simulink model "DZ_AC_ol"  (R2019b)
settings: Solver=VariableStepAuto  StartTime=0.0  StopTime=1  RelTol=1e-3
undefined symbols (not defined in the file): alfa_beta, beta, j, J, Lkm, Lks, np, omega, rad_to_rpm, Rr, Rs, T_1_amp, T_amp, Vmax
libraries: simulink x3
settings Model: Creator=denni  LastModifiedBy=denniszanutto

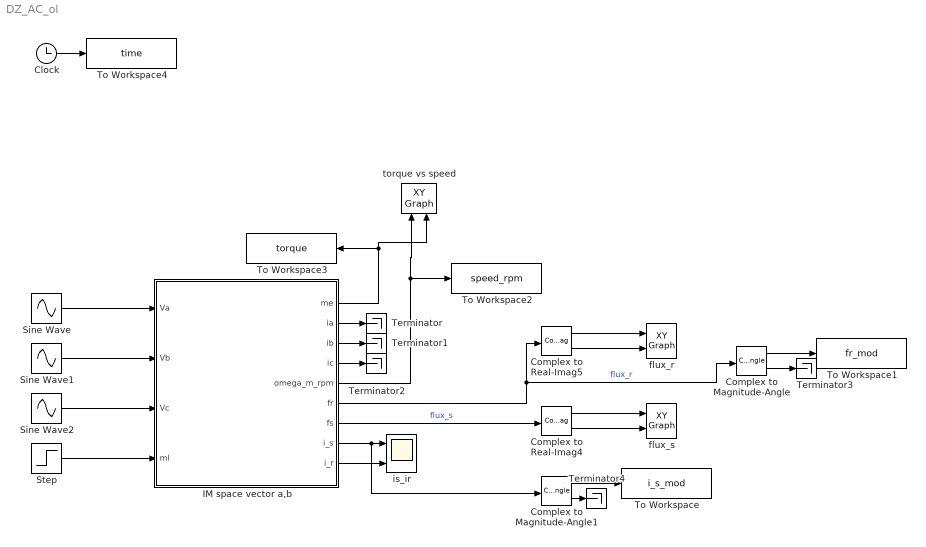
== system DZ_AC_ol ==
  Clock : Clock
  Complex to Magnitude-Angle : ComplexToMagnitudeAngle
  Complex to Magnitude-Angle1 : ComplexToMagnitudeAngle
  Complex to Real-Imag4 : ComplexToRealImag
  Complex to Real-Imag5 : ComplexToRealImag
  IM space vector a,b : Subsystem
  Sine Wave : Sin  Amplitude=Vmax  Frequency=omega  SampleTime=0
  Sine Wave1 : Sin  Amplitude=Vmax  Frequency=omega  Phase=-2*pi/3  SampleTime=0
  Sine Wave2 : Sin  Amplitude=Vmax  Frequency=omega  Phase=2*pi/3  SampleTime=0
  Step : Step  Time=0  After=0  SampleTime=0
  Terminator{,1..4} (5 alike) : Terminator
  To Workspace : ToWorkspace  VariableName=i_s_mod  SaveFormat=Timeseries  SampleTime=-1
  To Workspace1 : ToWorkspace  VariableName=fr_mod  SaveFormat=Timeseries  SampleTime=-1
  To Workspace2 : ToWorkspace  VariableName=speed_rpm  SaveFormat=Timeseries  SampleTime=-1
  To Workspace3 : ToWorkspace  VariableName=torque  SaveFormat=Timeseries  SampleTime=-1
  To Workspace4 : ToWorkspace  VariableName=time  SaveFormat=Timeseries  SampleTime=-1
  flux_r : simulink/Sinks/XY Graph  xmin=-3  xmax=3  ymin=-3  ymax=3  st=-1
  flux_s : simulink/Sinks/XY Graph  xmin=-3  xmax=3  ymin=-3  ymax=3  st=-1
  is_ir : Scope  NumInputPorts=2
  torque vs speed : simulink/Sinks/XY Graph  xmin=0  xmax=1300  ymin=-800  ymax=1200  st=-1
  wires:
  Step/1 -> IM space vector a,b/4(ml)
  Sine Wave/1 -> IM space vector a,b/1(Va)
  Sine Wave1/1 -> IM space vector a,b/2(Vb)
  Sine Wave2/1 -> IM space vector a,b/3(Vc)
  Complex to Real-Imag4/2 -> flux_s/2
  IM space vector a,b/7(fs) -> Complex to Real-Imag4/1  "flux_s"
  Complex to Real-Imag4/1 -> flux_s/1
  Complex to Real-Imag5/1 -> flux_r/1
  IM space vector a,b/6(fr) -> Complex to Real-Imag5/1, Complex to Magnitude-Angle/1  "flux_r"
  Complex to Real-Imag5/2 -> flux_r/2
  Complex to Magnitude-Angle/1 -> To Workspace1/1
  IM space vector a,b/8(i_s) -> Complex to Magnitude-Angle1/1, is_ir/1
  IM space vector a,b/9(i_r) -> is_ir/2
  IM space vector a,b/2(ia) -> Terminator/1
  IM space vector a,b/3(ib) -> Terminator1/1
  IM space vector a,b/4(ic) -> Terminator2/1
  IM space vector a,b/1("me ") -> torque vs speed/2, To Workspace3/1
  IM space vector a,b/5("omega_m_rpm ") -> To Workspace2/1, torque vs speed/1
  Complex to Magnitude-Angle/2 -> Terminator3/1
  Complex to Magnitude-Angle1/1 -> To Workspace/1
  Complex to Magnitude-Angle1/2 -> Terminator4/1
  Clock/1 -> To Workspace4/1

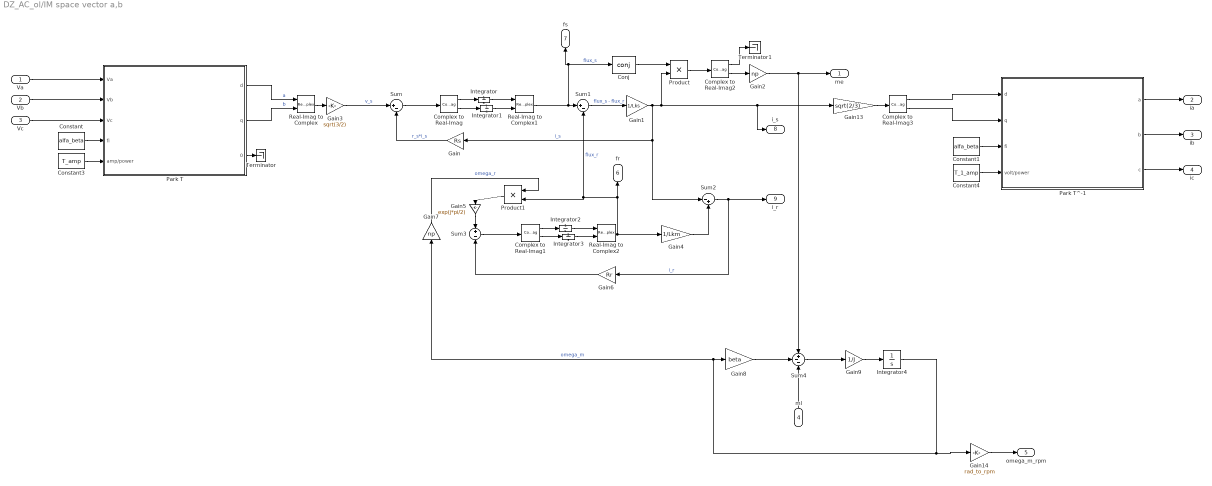
== system DZ_AC_ol/IM space vector a,b ==
  Va : Inport
  Vb : Inport  Port=2
  Vc : Inport  Port=3
  ml : Inport  Port=4
  Complex to Real-Imag{,1..3} (4 alike) : ComplexToRealImag
  Conj : Math  Operator=conj  SignedPower=off  SaturateOnIntegerOverflow=on
  Constant : Constant  Value=alfa_beta
  Constant1 : Constant  Value=alfa_beta
  Constant3 : Constant  Value=T_amp
  Constant4 : Constant  Value=T_1_amp
  Gain : Gain  Gain=Rs
  Gain1 : Gain  Gain=1/Lks
  Gain13 : Gain  Gain=sqrt(2/3)
  Gain14 : Gain  Gain=rad_to_rpm
  Gain2 : Gain  Gain=np
  Gain3 : Gain  Gain=sqrt(3/2)
  Gain4 : Gain  Gain=1/Lkm
  Gain5 : Gain  Gain=exp(j*pi/2)
  Gain6 : Gain  Gain=Rr
  Gain7 : Gain  Gain=np
  Gain8 : Gain  Gain=beta
  Gain9 : Gain  Gain=1/J
  Integrator{,1..4} (5 alike) : Integrator
  Park T : Subsystem
  Park T^-1 : Subsystem
  Product : Product
  Product1 : Product
  Real-Imag to Complex : RealImagToComplex
  Real-Imag to Complex1 : RealImagToComplex
  Real-Imag to Complex2 : RealImagToComplex
  Sum : Sum  Inputs=|+-
  Sum1 : Sum  Inputs=|+-
  Sum2 : Sum  Inputs=|-+
  Sum3 : Sum  Inputs=+-
  Sum4 : Sum  Inputs=+--
  Terminator : Terminator
  Terminator1 : Terminator
  "me " : Outport
  ia : Outport  Port=2
  ib : Outport  Port=3
  ic : Outport  Port=4
  "omega_m_rpm " : Outport  Port=5
  fr : Outport  Port=6
  fs : Outport  Port=7
  i_s : Outport  Port=8
  i_r : Outport  Port=9
  wires:
  Vc/1 -> Park T/3("Vc ")
  Constant/1 -> Park T/4(fi)
  Constant3/1 -> Park T/5("amp/power ")
  Park T/1(d) -> Real-Imag to Complex/1  "a"
  Park T/2("q ") -> Real-Imag to Complex/2  "b"
  Real-Imag to Complex/1 -> Gain3/1
  Sum/1 -> Complex to Real-Imag/1
  Complex to Real-Imag/1 -> Integrator/1
  Complex to Real-Imag/2 -> Integrator1/1
  Integrator/1 -> Real-Imag to Complex1/1
  Integrator1/1 -> Real-Imag to Complex1/2
  Gain/1 -> Sum/2  "r_s*i_s"
  Real-Imag to Complex1/1 -> fs/1, Conj/1, Sum1/1  "flux_s"
  Sum1/1 -> Gain1/1  "flux_s - flux_r"
  Gain1/1 -> Product/2, i_s/1, Gain13/1, Sum2/1, Gain/1  "i_s"
  Conj/1 -> Product/1
  Complex to Real-Imag1/1 -> Integrator2/1
  Complex to Real-Imag1/2 -> Integrator3/1
  Integrator2/1 -> Real-Imag to Complex2/1
  Integrator3/1 -> Real-Imag to Complex2/2
  Gain4/1 -> Sum2/2
  Real-Imag to Complex2/1 -> fr/1, Product1/2, Sum1/2, Gain4/1  "flux_r"
  Sum3/1 -> Complex to Real-Imag1/1
  Gain5/1 -> Sum3/1
  Product1/1 -> Gain5/1
  Gain6/1 -> Sum3/2
  Sum2/1 -> i_r/1, Gain6/1  "i_r"
  ml/1 -> Sum4/3
  Sum4/1 -> Gain9/1
  Gain9/1 -> Integrator4/1
  Product/1 -> Complex to Real-Imag2/1
  Integrator4/1 -> Gain14/1, Gain7/1, Gain8/1  "omega_m"
  Gain2/1 -> Sum4/1, "me "/1
  Va/1 -> Park T/1(Va)
  Vb/1 -> Park T/2(Vb)
  Gain8/1 -> Sum4/2
  Complex to Real-Imag2/2 -> Gain2/1
  Gain3/1 -> Sum/1  "v_s"
  Gain7/1 -> Product1/1  "omega_r"
  Gain13/1 -> Complex to Real-Imag3/1
  Complex to Real-Imag3/2 -> Park T^-1/2(q)
  Complex to Real-Imag3/1 -> Park T^-1/1(d)
  Constant1/1 -> Park T^-1/3(fi)
  Constant4/1 -> Park T^-1/4(volt/power)
  Park T^-1/1("a ") -> ia/1
  Park T^-1/2("b ") -> ib/1
  Park T^-1/3(c) -> ic/1
  Park T/3(0) -> Terminator/1
  Complex to Real-Imag2/1 -> Terminator1/1
  Gain14/1 -> "omega_m_rpm "/1

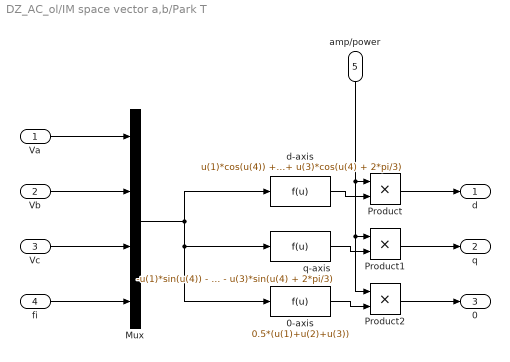
== system DZ_AC_ol/IM space vector a,b/Park T ==
  Va : Inport
  Vb : Inport  Port=2
  "Vc " : Inport  Port=3
  fi : Inport  Port=4
  "amp/power " : Inport  Port=5
  0-axis : Fcn  Expr=0.5*(u(1)+u(2)+u(3))
  Mux : Mux
  Product : Product
  Product1 : Product
  Product2 : Product
  "d-axis " : Fcn  Expr=u(1)*cos(u(4)) + u(2)*cos(u(4) -2*pi/3) + u(3)*cos(u(4) + 2*pi/3)
  q-axis : Fcn  Expr=-u(1)*sin(u(4)) - u(2)*sin(u(4) -2*pi/3) - u(3)*sin(u(4) + 2*pi/3)
  d : Outport
  "q " : Outport  Port=2
  0 : Outport  Port=3
  wires:
  fi/1 -> Mux/4
  Va/1 -> Mux/1
  Vb/1 -> Mux/2
  "Vc "/1 -> Mux/3
  Mux/1 -> "d-axis "/1, q-axis/1, 0-axis/1
  Product/1 -> d/1
  "d-axis "/1 -> Product/2
  Product1/1 -> "q "/1
  q-axis/1 -> Product1/2
  0-axis/1 -> Product2/2
  Product2/1 -> 0/1
  "amp/power "/1 -> Product2/1, Product1/1, Product/1

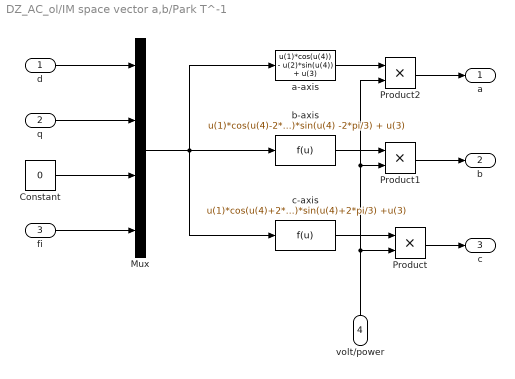
== system DZ_AC_ol/IM space vector a,b/Park T^-1 ==
  d : Inport
  q : Inport  Port=2
  fi : Inport  Port=3
  volt/power : Inport  Port=4
  Constant : Constant  Value=0
  Mux : Mux
  Product : Product
  Product1 : Product
  Product2 : Product
  "a-axis " : Fcn  Expr=u(1)*cos(u(4)) - u(2)*sin(u(4)) + u(3)
  b-axis : Fcn  Expr=u(1)*cos(u(4)-2*pi/3) - u(2)*sin(u(4) -2*pi/3) + u(3)
  c-axis : Fcn  Expr=u(1)*cos(u(4)+2*pi/3) -u(2)*sin(u(4)+2*pi/3) +u(3)
  "a " : Outport
  "b " : Outport  Port=2
  c : Outport  Port=3
  wires:
  fi/1 -> Mux/4
  d/1 -> Mux/1
  q/1 -> Mux/2
  Mux/1 -> c-axis/1, b-axis/1, "a-axis "/1
  Constant/1 -> Mux/3
  volt/power/1 -> Product2/2, Product1/2, Product/2
  c-axis/1 -> Product/1
  Product/1 -> c/1
  Product1/1 -> "b "/1
  b-axis/1 -> Product1/1
  Product2/1 -> "a "/1
  "a-axis "/1 -> Product2/1
